simulink model "perceptionBlockTest"  (R2025b)
settings: Solver=VariableStepAuto  StartTime=0.0  StopTime=10.0  RelTol=1e-3
settings Model: Creator=Ethan Dueck  LastModifiedBy=Ethan Dueck

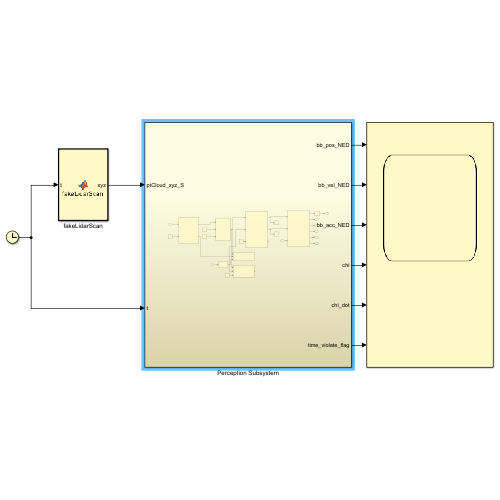
[thumbnail: Simulink's stored preview of the top-level diagram]
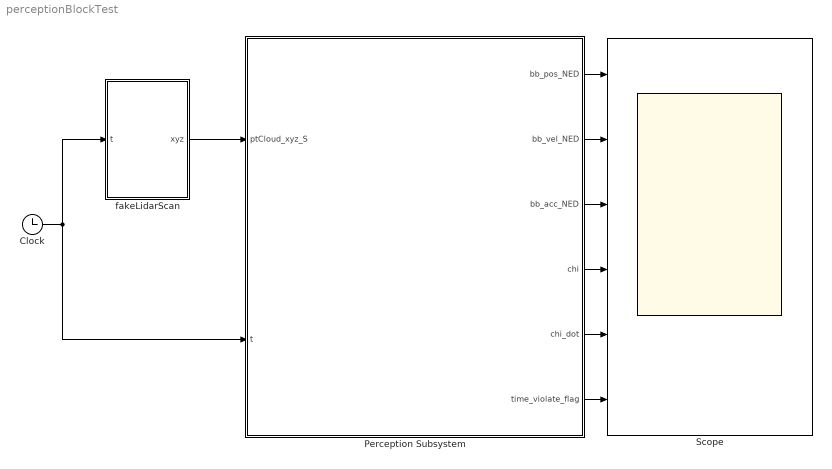
== system perceptionBlockTest ==
  Clock : Clock
  Perception Subsystem : Subsystem
  Scope : Scope  NumInputPorts=6
      settings: ActiveDisplayYMinimum=-0.60935310255606356  ActiveDisplayYMaximum=2.6534538943868244
  fakeLidarScan : MATLAB Function  TreatAsAtomicUnit=on
  wires:
  Clock/1 -> Perception Subsystem/2(t), fakeLidarScan/1(t)
  fakeLidarScan/1(xyz) -> Perception Subsystem/1(ptCloud_xyz_S)
  Perception Subsystem/1(bb_pos_NED) -> Scope/1
  Perception Subsystem/2(bb_vel_NED) -> Scope/2
  Perception Subsystem/3(bb_acc_NED) -> Scope/3
  Perception Subsystem/4(chi) -> Scope/4
  Perception Subsystem/5(chi_dot) -> Scope/5
  Perception Subsystem/6(time_violate_flag) -> Scope/6

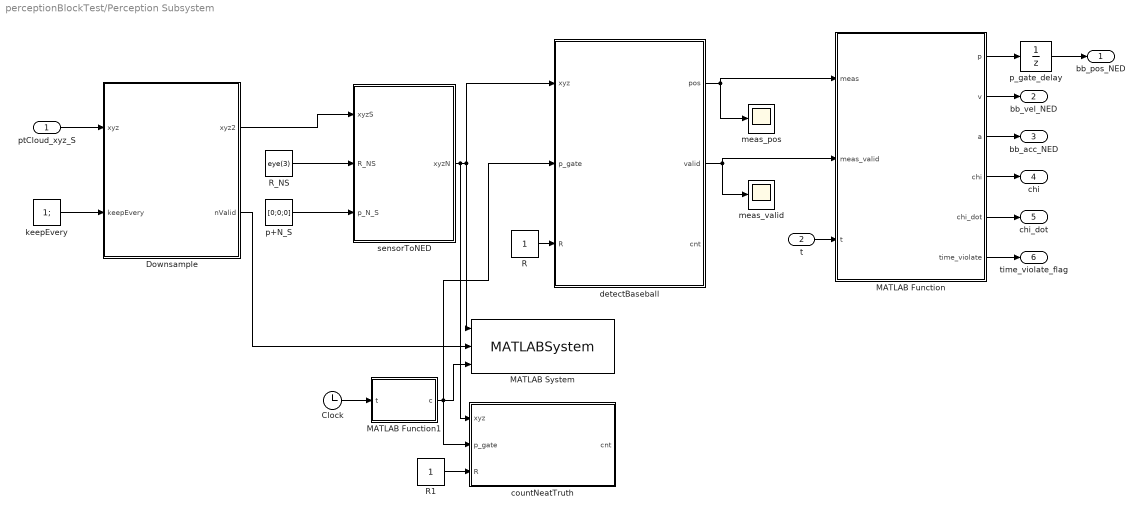
== system perceptionBlockTest/Perception Subsystem ==
  ptCloud_xyz_S : Inport
  t : Inport  Port=2
  Clock : Clock
  Downsample : MATLAB Function  TreatAsAtomicUnit=on
  MATLAB Function : MATLAB Function  TreatAsAtomicUnit=on
  MATLAB Function1 : MATLAB Function  TreatAsAtomicUnit=on
  MATLAB System : MATLABSystem  System=PointCloudViewer  PointSize=3  XLim=[0 60]  YLim=[-30 30]  ZLim=[-10 10]  Decimate=5  ShowDetection=on  SimulateUsing=Interpreted execution
      mask Type: PointCloudViewer
  R : Constant
  R1 : Constant
  R_NS : Constant  Value=eye(3)
  countNeatTruth : MATLAB Function  TreatAsAtomicUnit=on
  detectBaseball : MATLAB Function  TreatAsAtomicUnit=on
  keepEvery : Constant  Value=1;
  meas_pos : Scope
      settings: ActiveDisplayYMinimum=-16.997474195338938  ActiveDisplayYMaximum=39.269494336463588
  meas_valid : Scope
      settings: ActiveDisplayYMinimum=0.9  ActiveDisplayYMaximum=1.1  DataLoggingVariableName=ScopeData4
  p+N_S : Constant  Value=[0;0;0]
  p_gate_delay : UnitDelay  InitialCondition=[10; 0; -2]  SampleTime=-1  HasFrameUpgradeWarning=on
  sensorToNED : MATLAB Function  TreatAsAtomicUnit=on
  bb_pos_NED : Outport
  bb_vel_NED : Outport  Port=2
  bb_acc_NED : Outport  Port=3
  chi : Outport  Port=4
  chi_dot : Outport  Port=5
  time_violate_flag : Outport  Port=6
  wires:
  MATLAB Function/2(v) -> bb_vel_NED/1
  MATLAB Function/3(a) -> bb_acc_NED/1
  MATLAB Function/4(chi) -> chi/1
  MATLAB Function/5(chi_dot) -> chi_dot/1
  MATLAB Function/6(time_violate) -> time_violate_flag/1
  t/1 -> MATLAB Function/3(t)
  detectBaseball/2(valid) -> MATLAB Function/2(meas_valid), meas_valid/1
  R_NS/1 -> sensorToNED/2(R_NS)
  ptCloud_xyz_S/1 -> Downsample/1(xyz)
  Downsample/1(xyz2) -> sensorToNED/1(xyzS)
  keepEvery/1 -> Downsample/2(keepEvery)
  p+N_S/1 -> sensorToNED/3(p_N_S)
  MATLAB Function/1(p) -> p_gate_delay/1
  p_gate_delay/1 -> bb_pos_NED/1
  sensorToNED/1(xyzN) -> countNeatTruth/1(xyz), detectBaseball/1(xyz), MATLAB System/1
  Downsample/2(nValid) -> MATLAB System/2
  detectBaseball/1(pos) -> meas_pos/1, MATLAB Function/1(meas)
  Clock/1 -> MATLAB Function1/1(t)
  MATLAB Function1/1(c) -> detectBaseball/2(p_gate), countNeatTruth/2(p_gate), MATLAB System/3
  R/1 -> detectBaseball/3(R)
  R1/1 -> countNeatTruth/3(R)

== matlab function perceptionBlockTest/Perception Subsystem/sensorToNED ==
  data: xyzS input; xyzN output; R_NS input; p_N_S input
function xyzN = sensorToNED(xyzS, R_NS, p_N_S)
%#codegen
N = size(xyzS,1);
xyzN = zeros(N,3,'like',xyzS);

for i = 1:N
    p = xyzS(i,:).';
    if ~all(isfinite(p))
        xyzN(i,:) = [NaN NaN NaN];
    else
        q = R_NS*p + p_N_S;
        xyzN(i,:) = q.';
    end
end
end

== matlab function perceptionBlockTest/fakeLidarScan ==
  data: t input; xyz output
function xyz = fakeLidarScan(t)
%#codegen
% fakeLidarScan(t) - fixed-size 3D point cloud generator (11520x3)
% 16 channels x 720 azimuth samples = 11520 points/frame
%
% Frame: N, E, D where D is NEGATIVE-UP (your convention).
% This version guarantees a visible ball cluster every frame.

% -------------------- LiDAR config --------------------
nChan = int32(16);
nAz   = int32(720);
Npts  = 11520;              % 16*720

vUpDeg  = -5.0;             % slight down
vLowDeg = -35.0;            % more down

rangeMax = 100.0;           % m
minRange = 1.0;             % m

rotPerSec = 10.0;           % spins per second
yaw = 2*pi*rotPerSec*t;     % rad

% Sensor pose (NED)
pS = [0;0;0];               % at origin

% -------------------- Environment --------------------
% Ground plane at D=0 (since D negative is up, ground is 0)
D_ground = 0.0;

% Wall plane at N = 60 m
useWall = true;
N_wall  = 60.0;

% -------------------- Ball (truth) --------------------
ballCenter = [30; 0.5*t; -2.0];  % N,E,D (D negative-up)
ballRadius = 0.10;              % m

% Guaranteed visible returns (inject cluster)
injectBallCluster = true;
injectCount = int32(250);        % 50..500 typical
injectSigma = 0.03;              % m

% -------------------- Noise --------------------
rangeNoiseStd = 0.02;            % m
angNoiseStd   = 0.001;           % rad

% -------------------- Precompute vertical angles --------------------
vAngles = zeros(double(nChan),1);
for c = 1:double(nChan)
    frac = (double(c)-1.0) / (double(nChan)-1.0);
    vDeg = vUpDeg + frac*(vLowDeg - vUpDeg);
    vAngles(c) = vDeg * pi/180.0;
end

% -------------------- Allocate output (fixed-size) --------------------
xyz = zeros(Npts,3);

% -------------------- Generate scan --------------------
idx = 0;

for c = 1:double(nChan)
    v0 = vAngles(c);

    for k = 1:double(nAz)
        idx = idx + 1;

        % Azimuth (0..2pi) + yaw + small noise
        az = (double(k)-1.0) * (2*pi/double(nAz)) + yaw + angNoiseStd*randn();
        v  = v0 + angNoiseStd*randn();

        % Direction in a DOWN-positive convention first...
        dN = cos(v)*cos(az);
        dE = cos(v)*sin(az);
        dD_down = sin(v);     % positive down

        % Convert to your D-negative-up convention:
        dD = -dD_down;

        % ---- Intersect ground D = D_ground ----
        sGround = inf;
        if abs(dD) > 1e-6
            sGround = (D_ground - pS(3)) / dD;
            if sGround < minRange
                sGround = inf;
            end
        end

        % ---- Intersect wall N = N_wall ----
        sWall = inf;
        if useWall && abs(dN) > 1e-6
            sWall = (N_wall - pS(1)) / dN;
            if sWall < minRange
                sWall = inf;
            end
        end

        % nearest hit
        s = sGround;
        if sWall < s
            s = sWall;
        end

        if ~isfinite(s) || s > rangeMax
            s = rangeMax;
        end

        % range noise + clamp
        s = s + rangeNoiseStd*randn();
        if s < minRange, s = minRange; end
        if s > rangeMax, s = rangeMax; end

        p = pS + s*[dN; dE; dD];

        xyz(idx,:) = p.';
    end
end

% -------------------- Guaranteed ball cluster injection --------------------
if injectBallCluster
    % Overwrite a subset of rays with ball returns around ballCenter.
    % This guarantees countNearTruth > 0 and makes downstream perception work.
    for m = int32(1):injectCount
        ii = 1 + mod(double(m-1), Npts);
        xyz(ii,:) = (ballCenter + injectSigma*randn(3,1)).';
    end
else
    % If you later want to do "real" ray-ball intersection, add it here.
    % (We can implement a correct sphere intersection in your D convention.)
end

end

== matlab function perceptionBlockTest/Perception Subsystem/Downsample ==
  data: xyz input; xyz2 output; keepEvery input; nValid output
function [xyz2, nValid] = Downsample(xyz, keepEvery)
%#codegen
N = int32(size(xyz,1));          % should be 11520
xyz2 = zeros(double(N),3,'like',xyz);

nValid = int32(0);

k = int32(keepEvery);
if k < 1
    k = int32(1);
end

% Fill with NaNs (viewer will drop them; avoids axis blow-up)
nanv = cast(NaN,'like',xyz);
xyz2(:,:) = nanv;

j = int32(0);
for i = int32(1):k:N
    j = j + 1;
    xyz2(double(j),:) = xyz(double(i),:);
end

nValid = j;
end

== matlab function perceptionBlockTest/Perception Subsystem/MATLAB Function1 ==
  data: t input; c output
function c = ballTruth(t)
%#codegen
c = [30; 0.5*t; -2];
end

== matlab function perceptionBlockTest/Perception Subsystem/countNeatTruth ==
  data: xyz input; cnt output; p_gate input; R input
function cnt = countNearTruth(xyz, p_gate, R)
%#codegen
cnt = int32(0);
R2 = double(R)*double(R);

N = size(xyz,1);
for i = 1:N
    n = xyz(i,1); e = xyz(i,2); d = xyz(i,3);
    if ~isfinite(n) || ~isfinite(e) || ~isfinite(d)
        continue;
    end
    dn = n - p_gate(1);
    de = e - p_gate(2);
    dd = d - p_gate(3);
    if (dn*dn + de*de + dd*dd) <= R2
        cnt = cnt + 1;
    end
end
end

== matlab function perceptionBlockTest/Perception Subsystem/detectBaseball ==
  data: xyz input; pos output; valid output; cnt output; p_gate input; R input
function [pos, valid, cnt] = detectBallSphereGate(xyz, p_gate, R)
%#codegen
pos   = zeros(3,1);
valid = false;
cnt   = int32(0);

R2 = double(R)*double(R);
s  = zeros(3,1);

N = size(xyz,1);
for i = 1:N
    n = xyz(i,1); e = xyz(i,2); d = xyz(i,3);
    if ~isfinite(n) || ~isfinite(e) || ~isfinite(d)
        continue;
    end

    dn = n - p_gate(1);
    de = e - p_gate(2);
    dd = d - p_gate(3);

    if (dn*dn + de*de + dd*dd) <= R2
        cnt = cnt + 1;
        s = s + [n; e; d];
    end
end

if cnt >= 5
    pos = s / double(cnt);
    valid = true;
end
end

== matlab function perceptionBlockTest/Perception Subsystem/MATLAB Function ==
  data: meas input; p output; meas_valid input; t input; v output; a output; chi output; chi_dot output; time_violate output
function [p,v,a,chi,chi_dot,time_violate] = trackBaseball(meas, meas_valid, t)
%#codegen

persistent p_hat v_hat a_hat t_last t_meas_last init

if isempty(init)
    p_hat = zeros(3,1);
    v_hat = zeros(3,1);
    a_hat = zeros(3,1);
    t_last = t;
    t_meas_last = t;     % <-- avoid -Inf
    init = true;
end

% Guard against time going backwards or being constant
dt_raw = t - t_last;
if ~isfinite(dt_raw) || dt_raw <= 0
    dt = 1e-3;
else
    dt = dt_raw;
end
t_last = t;

% prediction
p_hat = p_hat + v_hat*dt + 0.5*a_hat*(dt*dt);
v_hat = v_hat + a_hat*dt;

% update (alpha-beta-gamma)
alpha = 0.7; beta = 0.2; gamma = 0.05;

meas_ok = meas_valid && all(isfinite(meas(:)));

if meas_ok
    r = meas - p_hat;
    p_hat = p_hat + alpha*r;
    v_hat = v_hat + (beta/dt)*r;
    a_hat = a_hat + (2*gamma/(dt*dt))*r;
    t_meas_last = t;
end

% outputs
p = p_hat; v = v_hat; a = a_hat;

% chi, chi_dot in NED horizontal plane (N=x, E=y)
vn = v(1); ve = v(2);
an = a(1); ae = a(2);

chi = atan2(ve, vn);
chi_dot = (vn*ae - ve*an) / (vn*vn + ve*ve + 1e-6);

% flag if no measurement for too long
age = t - t_meas_last;
if ~isfinite(age) || age < 0
    age = 0;
end
time_violate = age > 0.25;
end
